simulink model "viterby"  (R2020b)
settings: Solver=FixedStepAuto  StartTime=0.0  StopTime=8  FixedStep=0.1  RelTol=1e-3
libraries: simulink_extras x4, commutil2 x2, hdlsllib x1
settings Model: Creator=user  LastModifiedBy=user
settings SFSimCC: CustomCodeUndefinedFunction=UseInterfaceOnly

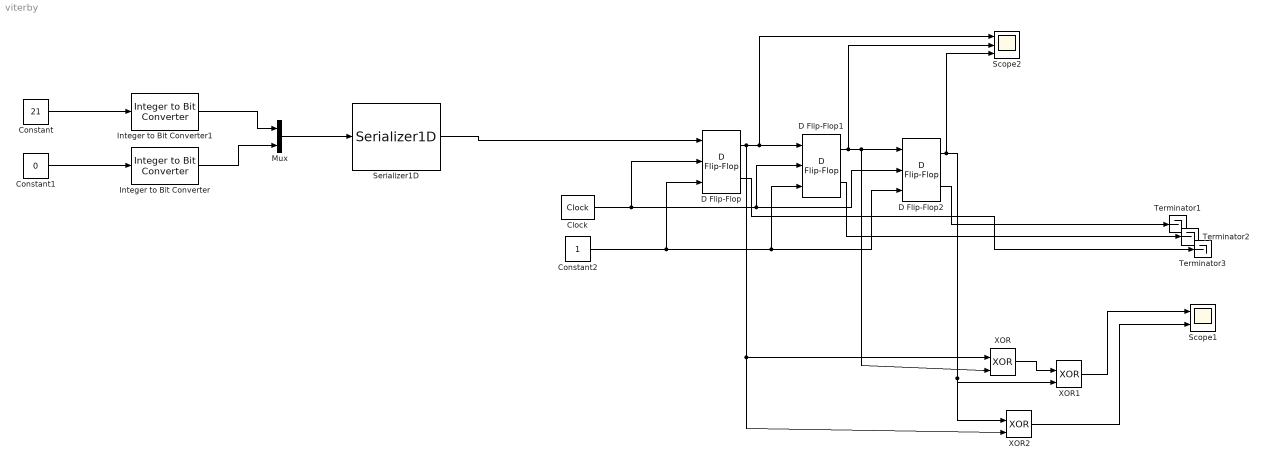
== system viterby ==
  Clock : simulink_extras/Flip Flops/Clock  period=1
  Constant : Constant  Value=21
  Constant1 : Constant  Value=0
  Constant2 : Constant  OutDataTypeStr=boolean
  D Flip-Flop : simulink_extras/Flip Flops/D Flip-Flop
  D Flip-Flop1 : simulink_extras/Flip Flops/D Flip-Flop
  D Flip-Flop2 : simulink_extras/Flip Flops/D Flip-Flop
  Integer to Bit Converter : commutil2/Integer to Bit Converter  nbits=2  signedInputValues=Unsigned  bitOrder=MSB first  outDtype=boolean
  Integer to Bit Converter1 : commutil2/Integer to Bit Converter  nbits=5  signedInputValues=Unsigned  bitOrder=MSB first  outDtype=boolean
  Mux : Mux  Inputs=2
  Scope1 : Scope  NumInputPorts=2
  Scope2 : Scope  NumInputPorts=3
  Serializer1D : hdlsllib/HDL Operations/Serializer1D  Ratio=7  IdleCycles=0  validIn=off  startOut=off  validOut=off  inputDataDimensions=-1  inputSampleTime=7  inputSignalType=auto
      settings: SourceProductBaseCode=SL
  Terminator1 : Terminator
  Terminator2 : Terminator
  Terminator3 : Terminator
  XOR : Logic  Operator=XOR  IconShape=distinctive  AllPortsSameDT=off  OutDataTypeStr=boolean
  XOR1 : Logic  Operator=XOR  IconShape=distinctive  AllPortsSameDT=off  OutDataTypeStr=boolean
  XOR2 : Logic  Operator=XOR  IconShape=distinctive  AllPortsSameDT=off  OutDataTypeStr=boolean
  wires:
  Constant/1 -> Integer to Bit Converter1/1
  Constant1/1 -> Integer to Bit Converter/1
  Integer to Bit Converter/1 -> Mux/2
  Mux/1 -> Serializer1D/1
  Serializer1D/1 -> D Flip-Flop/1
  D Flip-Flop1/1 -> Scope2/2, XOR/2, D Flip-Flop2/1
  D Flip-Flop2/1 -> Scope2/3, XOR1/2, XOR2/1
  D Flip-Flop/1 -> XOR/1, XOR2/2, Scope2/1, D Flip-Flop1/1
  Clock/1 -> D Flip-Flop/2, D Flip-Flop1/2, D Flip-Flop2/2
  D Flip-Flop2/2 -> Terminator1/1
  D Flip-Flop1/2 -> Terminator2/1
  D Flip-Flop/2 -> Terminator3/1
  Integer to Bit Converter1/1 -> Mux/1
  XOR/1 -> XOR1/1
  XOR1/1 -> Scope1/1
  XOR2/1 -> Scope1/2
  Constant2/1 -> D Flip-Flop/3, D Flip-Flop1/3, D Flip-Flop2/3
